simulink model "Single_Phase_Induction_Motor"  (R2021b)
settings: Solver=ode23s  StartTime=0.0  StopTime=10  MaxStep=1e-4  RelTol=1e-3
libraries: spsACVoltageSourceLib x1, spsSinglePhaseAsynchronousMachineLib x1, spspowerguiLib x1
settings Model: Creator=praveen  LastModifiedBy=rajshah
settings SolverCC: ZeroCrossAlgorithm=Adaptive
settings DebuggingCC: IgnoredZcDiagnostic=none

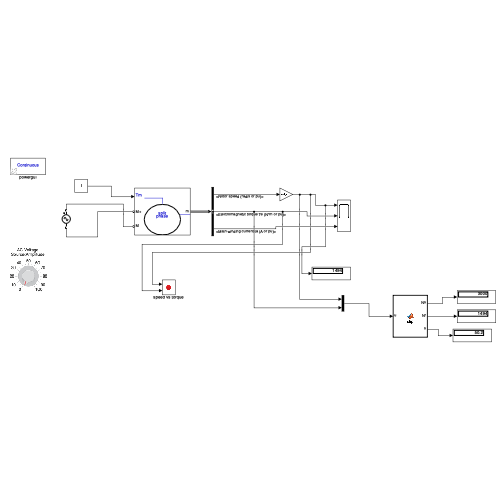
[thumbnail: Simulink's stored preview of the top-level diagram]
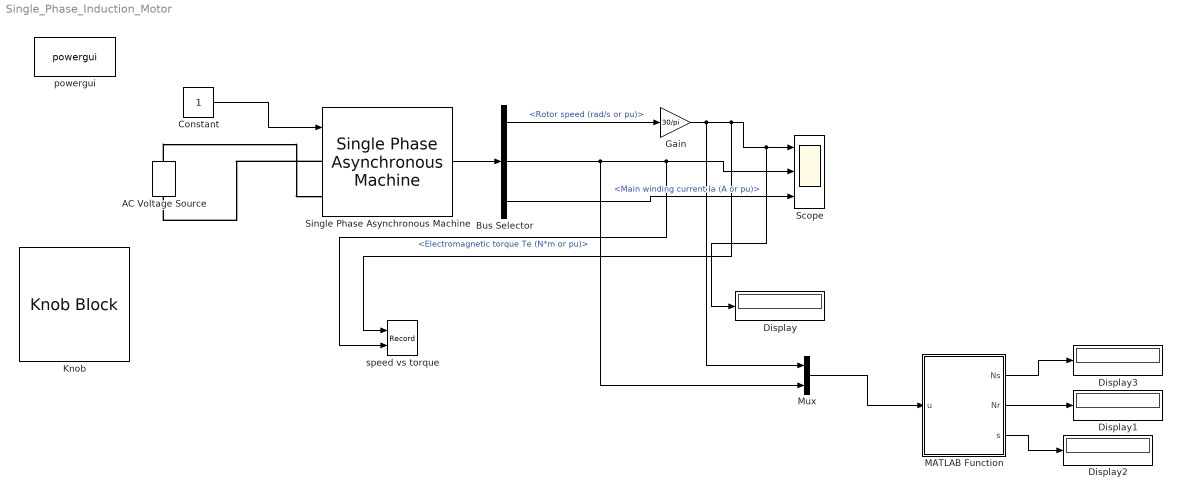
== system Single_Phase_Induction_Motor ==
  AC Voltage Source : spsACVoltageSourceLib/AC Voltage Source  Amplitude=-330  Phase=0  Frequency=50  SampleTime=0  Measurements=None  BusType=swing  Pref=10e3  Qref=0  Qmin=-inf  Qmax=+inf
  Bus Selector : BusSelector  OutputSignals=Mechanical.Rotor speed (rad/s or pu),Mechanical.Electromagnetic torque Te (N*m or pu),Stator measurements.Main winding current Ia (A or pu)
  Constant : Constant
  Display{,1..3} (4 alike) : Display
  Gain : Gain  Gain=30/pi
  Knob : KnobBlock
  MATLAB Function : MATLAB Function  TreatAsAtomicUnit=on
  Mux : Mux  Inputs=2
  Scope : Scope  NumInputPorts=3
  Single Phase Asynchronous Machine : spsSinglePhaseAsynchronousMachineLib/Single Phase Asynchronous Machine  MechanicalLoad=Torque Tm  UNITS=SI  MachineType=Split Phase  MeasurementBus=off  NominalParameters="[ .25*746  220 50]"  MainWindingStator="[2.02  7.4e-3]"  MainWindingRotor="[4.12  5.6e-3]"  MutualInductance=0.1772  AuxiliaryWinding="[7.14  8.5e-3]"  Mechanical="[0.0146  0  2 1.18]"  CapacitorStart="[2  254.7e-6]"  CapacitorRun="[18  21.1e-6]"  DisconnectionSpeed=75  InitialSpeed=0  DataType=SI  TsPowergui=0  TsBlock=-1
      settings: SourceProductBaseCode=PS
  powergui : spspowerguiLib/powergui  Priority=1  SimulationMode=Continuous  SampleTime=50e-6  frequency=60  Iterations=50  frequencyindice=50  Pbase=100e6  ErrMax=1e-4  UnitsV=kV  UnitsW=MW  buscounter=0  FunctionMessages=off  echomessages=off  EnableUseOfTLC=off  CurrentSourceSwitches=off  DisableSnubberDevices=off  DisableRonSwitches=off  DisableVfSwitches=off  DisplayEquations=off  AutomaticDiscreteSolvers=off  SolverType=Tustin/Backward Euler (TBE)  Interpol=off  ExternalGateDelay=off  methode=off  Ts=100  x0status=blocks  SPID=on  SwTol=0  HookPort=off  NonlinearTolerance=1e-4  nMaxIteration=100  ContinueOnMaxIteration=off  RestoreLinks=warning  ResistiveCurrentMeasurement=off  Frange=[0:2:500]  Ylog=off  Xlog=on  ShowGrid=off  save=off  variable=ZData  structure=0  ZoomFFT=off  StartTime=0.0  cycles=1  DisplayStyle=1  fundamental=60  FreqAxis=off  MaxFrequency=1000  frequencyindicesteady=1  RmsSteady=1  display=off
  speed vs torque : Record  FileSettingsInternal="{\"entries\":[{\"content\":{\"excelSettings\":{\"content\":{},\"type\":\"Streamout.ExcelSettings\"}},\"type\":\"Streamout.FileSettingStorage\",\"uuid\":\"ba92620f-005a-401d-b11c-2729753bf45f\"}],\"packageUris\":[\"http://schema.mathworks.com/mf0/streamout_blocks/R2020a\"],\"version\":\"1.0\"}"  Layout=[1 1]  SignalsInternal="{\"entries\":[{\"content\":{\"signals\":[{\"content\":{\"blockPath\":[\"Single_Phase_Induction_Motor/speed vs torque\"],\"channel\":[],\"dimensions\":[1],\"domain\":\"Single_Phase_Induction_Motor/speed vs torque\",\"lineColor\":\"#a2142f\",\"plots\":[1],\"port\":1,\"sid\":[\"\"],\"signalID\":1580,\"signalName\":\"Gain\"},\"type\":\"RecordBlkView.Signal\",\"uuid\":\"d4f74786-4319-4a99-9dad-b994138e7e76\"},{\"content\":{\"blockPath\":[\"Single_Phase_Induction_Motor/speed vs torque\"],\"channel\":[],\"dimensions\":[1],\"domain\":\"Single_Phase_Induction_Motor/speed vs torque\",\"lineColor\":\"#139fff\",\"plots\":[1],\"port\":2,\"sid\":[\"\"],\"signalID\":1584,\"signalName\":\"<Electromagnetic torque Te (N*m or pu)>\"},\"type\":\"RecordBlkView.Signal\",\"uuid\":\"a3273b94-7af8-40d2-87c9-c5802854709a\"}]},\"type\":\"RecordBlkView.InputSignals\",\"uuid\":\"b4f7e7c0-42fe-4531-ba4f-9044215f919f\"}],\"packageUris\":[\"http://schema.mathworks.com/mf0/streamout_blocks/R2020a\"],\"version\":\"1.0\"}"  VisualizationBindings="{\"xyplotplugin\":{\"info\":[{\"series\":[{\"bindingParametersList\":[{\"parameter\":\"X-Axis\",\"signalID\":1580,\"signalName\":\"Gain\"},{\"parameter\":\"Y-Axis\",\"signalID\":1584,\"signalName\":\"<Electromagnetic torque Te (N*m or pu)>\"}],\"seriesID\":5045}],\"subplotID\":1}]}}"  CompatibilityTag=XY  st=1e-4
  wires:
  Constant/1 -> Single Phase Asynchronous Machine/1
  Single Phase Asynchronous Machine/1 -> Bus Selector/1
  Bus Selector/3 -> Scope/3  "<Main winding current Ia (A or pu)>"
  Bus Selector/1 -> Gain/1  "<Rotor speed (rad/s or pu)>"
  Gain/1 -> Mux/1, speed vs torque/1, Display/1, Scope/1
  Bus Selector/2 -> Mux/2, speed vs torque/2, Scope/2  "<Electromagnetic torque Te (N*m or pu)>"
  Mux/1 -> MATLAB Function/1(u)
  MATLAB Function/1(Ns) -> Display3/1
  MATLAB Function/2(Nr) -> Display1/1
  MATLAB Function/3(s) -> Display2/1
  connections:
  Single Phase Asynchronous Machine/LConn1 -- AC Voltage Source/LConn1
  AC Voltage Source/RConn1 -- Single Phase Asynchronous Machine/LConn2

== matlab function Single_Phase_Induction_Motor/MATLAB Function ==
  data: Ns output; Nr output; u input; s output
function [Ns,Nr,s] = slip(u)
Ns= (2*50*60)/2;
s=((Ns-u(1))/Ns)*100;
Nr= u(1);
end
